simulink model "InversorTrifasico"  (R2022b)
settings: Solver=VariableStepAuto  StartTime=0.0  StopTime=3  MaxStep=0.00001  RelTol=1e-3
libraries: spsIGBTDiodeLib x6, spsVoltageMeasurementLib x3, spsSeriesRLCBranchLib x3, spsMeanLib x2, spsRMSLib x2, spsDCVoltageSourceLib x1, sps_lib x1
settings Model: Creator=mique  LastModifiedBy=ramuj

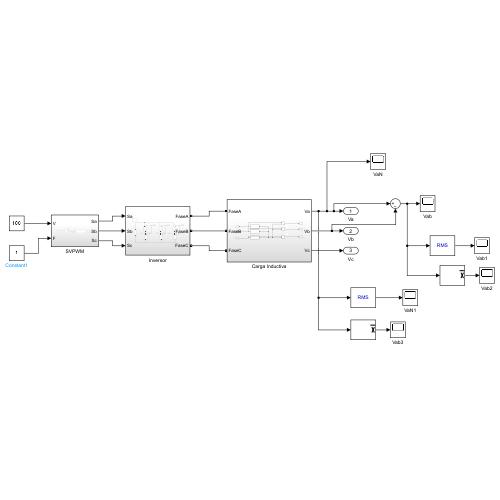
[thumbnail: Simulink's stored preview of the top-level diagram]
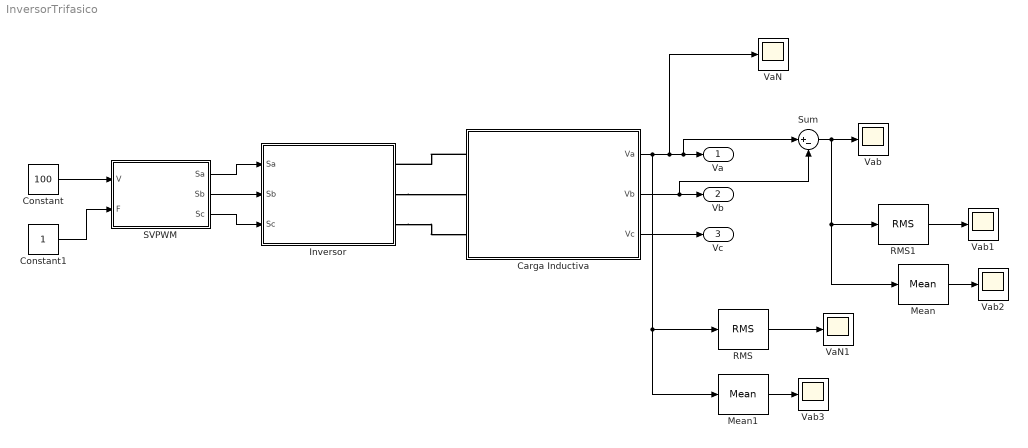
== system InversorTrifasico ==
  Carga Inductiva : Subsystem
  Constant : Constant  Value=100
  Constant1 : Constant
  Inversor : Subsystem
  Mean : spsMeanLib/Mean  Freq=60  Vinit=0  Ts=0
  Mean1 : spsMeanLib/Mean  Freq=60  Vinit=0  Ts=0
  RMS : spsRMSLib/RMS  TrueRMS=on  Freq=60  RMSInit=120  Ts=0
  RMS1 : spsRMSLib/RMS  TrueRMS=on  Freq=60  RMSInit=120  Ts=0
  SVPWM : Subsystem
  Sum : Sum  Inputs=|+-
  VaN : Scope
  VaN1 : Scope
  Vab{,1..3} (4 alike) : Scope
  Va : Outport
  Vb : Outport  Port=2
  Vc : Outport  Port=3
  wires:
  Carga Inductiva/2(Vb) -> Sum/2, Vb/1
  Carga Inductiva/3(Vc) -> Vc/1
  SVPWM/1(Sa) -> Inversor/1(Sa)
  SVPWM/2(Sb) -> Inversor/2(Sb)
  SVPWM/3(Sc) -> Inversor/3(Sc)
  Constant/1 -> SVPWM/1(V)
  Constant1/1 -> SVPWM/2(F)
  Sum/1 -> Mean/1, RMS1/1, Vab/1
  RMS/1 -> VaN1/1
  RMS1/1 -> Vab1/1
  Mean/1 -> Vab2/1
  Carga Inductiva/1(Va) -> Mean1/1, RMS/1, VaN/1, Sum/1, Va/1
  Mean1/1 -> Vab3/1
  connections:
  Carga Inductiva/LConn1 -- Inversor/RConn1
  Inversor/RConn2 -- Carga Inductiva/LConn2
  Inversor/RConn3 -- Carga Inductiva/LConn3

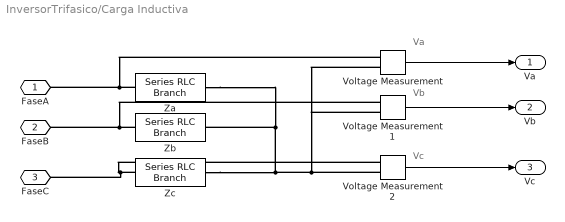
== system InversorTrifasico/Carga Inductiva ==
  note: Va
  note: Vb
  note: Vc
  Voltage Measurement : spsVoltageMeasurementLib/Voltage Measurement  PhasorSimulation=off  OutputType=Complex  PSBequivalent=0
  Voltage Measurement1 : spsVoltageMeasurementLib/Voltage Measurement  PhasorSimulation=off  OutputType=Complex  PSBequivalent=0
  Voltage Measurement2 : spsVoltageMeasurementLib/Voltage Measurement  PhasorSimulation=off  OutputType=Complex  PSBequivalent=0
  Za : spsSeriesRLCBranchLib/Series RLC Branch  LConnTagsString=__new0  RConnTagsString=__new0  BranchType=RL  Resistance=1e-3  Inductance=21e-3  SetiL0=off  InitialCurrent=0  Capacitance=1e-6  Setx0=off  InitialVoltage=0  Measurements=None
  Zb : spsSeriesRLCBranchLib/Series RLC Branch  LConnTagsString=__new0  RConnTagsString=__new0  BranchType=RL  Resistance=1e-3  Inductance=21e-3  SetiL0=off  InitialCurrent=0  Capacitance=1e-6  Setx0=off  InitialVoltage=0  Measurements=None
  Zc : spsSeriesRLCBranchLib/Series RLC Branch  LConnTagsString=__new0  RConnTagsString=__new0  BranchType=RL  Resistance=1e-3  Inductance=21e-3  SetiL0=off  InitialCurrent=0  Capacitance=1e-6  Setx0=off  InitialVoltage=0  Measurements=None
  FaseA : PMIOPort  Side=Left
  FaseB : PMIOPort  Port=2  Side=Left
  FaseC : PMIOPort  Port=3  Side=Left
  Va : Outport
  Vb : Outport  Port=2
  Vc : Outport  Port=3
  wires:
  Voltage Measurement/1 -> Va/1
  Voltage Measurement1/1 -> Vb/1
  Voltage Measurement2/1 -> Vc/1
  connections:
  Voltage Measurement1/LConn1 -- FaseB/RConn1 -- Zb/LConn1
  Voltage Measurement/LConn1 -- Za/LConn1 -- FaseA/RConn1
  Zc/RConn1 -- Voltage Measurement1/LConn2 -- Voltage Measurement/LConn2 -- Voltage Measurement2/LConn2 -- Za/RConn1 -- Zb/RConn1
  Voltage Measurement2/LConn1 -- Zc/LConn1 -- FaseC/RConn1

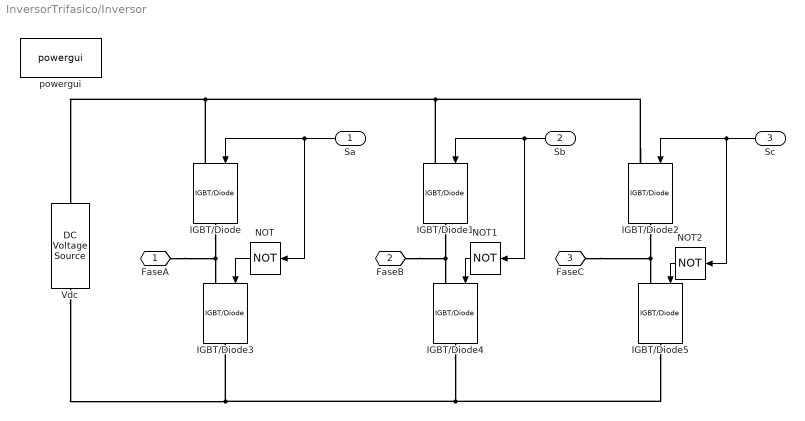
== system InversorTrifasico/Inversor ==
  Sa : Inport
  Sb : Inport  Port=2
  Sc : Inport  Port=3
  IGBT/Diode{,1..5} (6 alike) : spsIGBTDiodeLib/IGBT//Diode  Ron=1e-3  Rs=1e5  Cs=inf  Measurements=off
  NOT : Logic  Operator=NOT  IconShape=distinctive  AllPortsSameDT=off  OutDataTypeStr=boolean
  NOT1 : Logic  Operator=NOT  IconShape=distinctive  AllPortsSameDT=off  OutDataTypeStr=boolean
  NOT2 : Logic  Operator=NOT  IconShape=distinctive  AllPortsSameDT=off  OutDataTypeStr=boolean
  Vdc : spsDCVoltageSourceLib/DC Voltage Source  Amplitude=200  Measurements=None
  powergui : sps_lib/powergui  Priority=1  SimulationMode=Continuous  SampleTime=50e-6  frequency=60  Iterations=50  frequencyindice=0  Pbase=100e6  ErrMax=1e-4  UnitsV=kV  UnitsW=MW  buscounter=0  FunctionMessages=off  echomessages=off  EnableUseOfTLC=off  CurrentSourceSwitches=off  DisableSnubberDevices=off  DisableRonSwitches=off  DisableVfSwitches=off  DisplayEquations=off  AutomaticDiscreteSolvers=off  SolverType=Tustin/Backward Euler (TBE)  Interpol=off  ExternalGateDelay=off  methode=off  Ts=100  x0status=blocks  SPID=on  SwTol=0  HookPort=off  NonlinearTolerance=1e-4  nMaxIteration=100  ContinueOnMaxIteration=off  RestoreLinks=warning  ResistiveCurrentMeasurement=off  Frange=[0:2:500]  Ylog=off  Xlog=on  ShowGrid=off  save=off  variable=ZData  structure=0  ZoomFFT=off  StartTime=0.0  cycles=1  DisplayStyle=1  fundamental=60  FreqAxis=off  MaxFrequency=1000  frequencyindicesteady=1  RmsSteady=1  display=off
  FaseA : PMIOPort  Side=Right
  FaseB : PMIOPort  Port=2  Side=Right
  FaseC : PMIOPort  Port=3  Side=Right
  wires:
  Sa/1 -> IGBT/Diode/1, NOT/1
  NOT1/1 -> IGBT/Diode4/1
  Sb/1 -> IGBT/Diode1/1, NOT1/1
  NOT2/1 -> IGBT/Diode5/1
  Sc/1 -> IGBT/Diode2/1, NOT2/1
  NOT/1 -> IGBT/Diode3/1
  connections:
  Vdc/LConn1 -- IGBT/Diode3/RConn1 -- IGBT/Diode4/RConn1 -- IGBT/Diode5/RConn1
  IGBT/Diode2/RConn1 -- FaseC/RConn1 -- IGBT/Diode5/LConn1
  IGBT/Diode/LConn1 -- IGBT/Diode2/LConn1 -- IGBT/Diode1/LConn1 -- Vdc/RConn1
  IGBT/Diode/RConn1 -- FaseA/RConn1 -- IGBT/Diode3/LConn1
  IGBT/Diode1/RConn1 -- FaseB/RConn1 -- IGBT/Diode4/LConn1

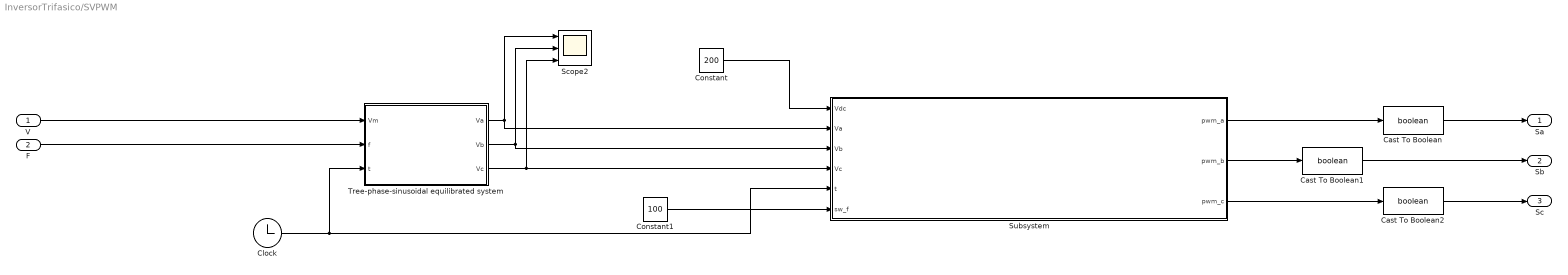
== system InversorTrifasico/SVPWM ==
  V : Inport
  F : Inport  Port=2
  Cast To Boolean : DataTypeConversion  OutDataTypeStr=boolean  SaturateOnIntegerOverflow=off  RndMeth=Floor
  Cast To Boolean1 : DataTypeConversion  OutDataTypeStr=boolean  SaturateOnIntegerOverflow=off  RndMeth=Floor
  Cast To Boolean2 : DataTypeConversion  OutDataTypeStr=boolean  SaturateOnIntegerOverflow=off  RndMeth=Floor
  Clock : Clock
  Constant : Constant  Value=200
  Constant1 : Constant  Value=100
  Scope2 : Scope  NumInputPorts=3
  Subsystem : Subsystem
  Tree-phase-sinusoidal equilibrated system : Subsystem
  Sa : Outport
  Sb : Outport  Port=2
  Sc : Outport  Port=3
  wires:
  Subsystem/1(pwm_a) -> Cast To Boolean/1
  Tree-phase-sinusoidal equilibrated system/3(Vc) -> Scope2/3, Subsystem/4(Vc)
  V/1 -> Tree-phase-sinusoidal equilibrated system/1(Vm)
  Subsystem/2(pwm_b) -> Cast To Boolean1/1
  F/1 -> Tree-phase-sinusoidal equilibrated system/2(f)
  Constant1/1 -> Subsystem/6(sw_f)
  Subsystem/3(pwm_c) -> Cast To Boolean2/1
  Clock/1 -> Tree-phase-sinusoidal equilibrated system/3(t), Subsystem/5(t)
  Tree-phase-sinusoidal equilibrated system/2(Vb) -> Scope2/2, Subsystem/3(Vb)
  Tree-phase-sinusoidal equilibrated system/1(Va) -> Scope2/1, Subsystem/2(Va)
  Cast To Boolean/1 -> Sa/1
  Cast To Boolean1/1 -> Sb/1
  Constant/1 -> Subsystem/1(Vdc)
  Cast To Boolean2/1 -> Sc/1

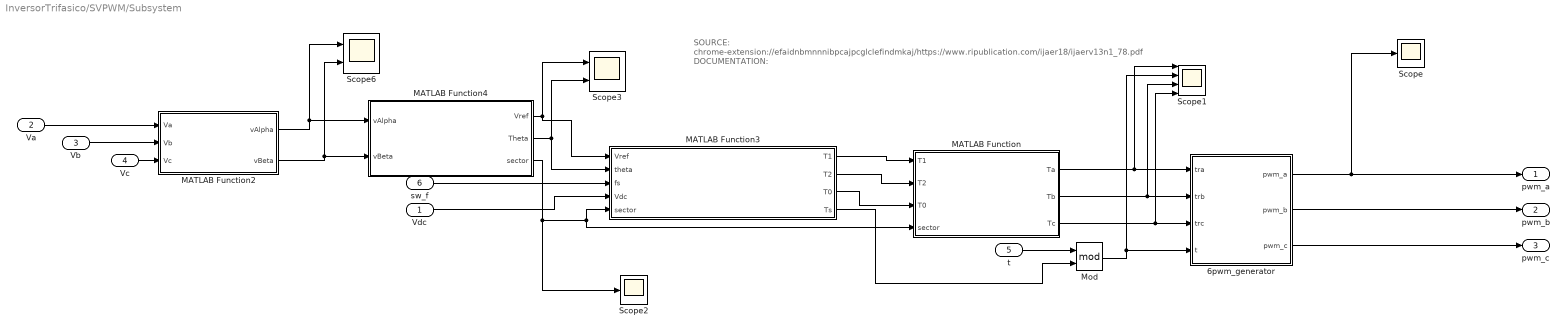
== system InversorTrifasico/SVPWM/Subsystem ==
  note: SOURCE:
      | chrome-extension://efaidnbmnnnibpcajpcglclefindmkaj/https://www.ripublication.com/ijaer18/ijaerv13n1_78.pdf
      | DOCUMENTATION:
  Vdc : Inport
  Va : Inport  Port=2
  Vb : Inport  Port=3
  Vc : Inport  Port=4
  t : Inport  Port=5
  sw_f : Inport  Port=6
  6pwm_generator : Subsystem
  MATLAB Function : MATLAB Function  TreatAsAtomicUnit=on
  MATLAB Function2 : MATLAB Function  TreatAsAtomicUnit=on
  MATLAB Function3 : MATLAB Function  TreatAsAtomicUnit=on
  MATLAB Function4 : MATLAB Function  TreatAsAtomicUnit=on
  Mod : Math  Operator=mod
  Scope : Scope
  Scope1 : Scope  NumInputPorts=4
  Scope2 : Scope
  Scope3 : Scope  NumInputPorts=2
  Scope6 : Scope  NumInputPorts=2
  pwm_a : Outport
  pwm_b : Outport  Port=2
  pwm_c : Outport  Port=3
  wires:
  MATLAB Function4/3(sector) -> Scope2/1, MATLAB Function/4(sector), MATLAB Function3/5(sector)
  MATLAB Function3/1(T1) -> MATLAB Function/1(T1)
  MATLAB Function2/2(vBeta) -> Scope6/2, MATLAB Function4/2(vBeta)
  MATLAB Function4/2(Theta) -> MATLAB Function3/2(theta), Scope3/2
  MATLAB Function4/1(Vref) -> MATLAB Function3/1(Vref), Scope3/1
  MATLAB Function3/3(T0) -> MATLAB Function/3(T0)
  MATLAB Function3/2(T2) -> MATLAB Function/2(T2)
  Vdc/1 -> MATLAB Function3/4(Vdc)
  MATLAB Function2/1(vAlpha) -> MATLAB Function4/1(vAlpha), Scope6/1
  MATLAB Function/2(Tb) -> Scope1/3, 6pwm_generator/2(trb)
  6pwm_generator/3(pwm_c) -> pwm_c/1
  MATLAB Function/1(Ta) -> Scope1/1, 6pwm_generator/1(tra)
  sw_f/1 -> MATLAB Function3/3(fs)
  MATLAB Function/3(Tc) -> Scope1/4, 6pwm_generator/3(trc)
  Vb/1 -> MATLAB Function2/2(Vb)
  Va/1 -> MATLAB Function2/1(Va)
  Vc/1 -> MATLAB Function2/3(Vc)
  6pwm_generator/1(pwm_a) -> Scope/1, pwm_a/1
  6pwm_generator/2(pwm_b) -> pwm_b/1
  t/1 -> Mod/1
  Mod/1 -> Scope1/2, 6pwm_generator/4(t)
  MATLAB Function3/4(Ts) -> Mod/2

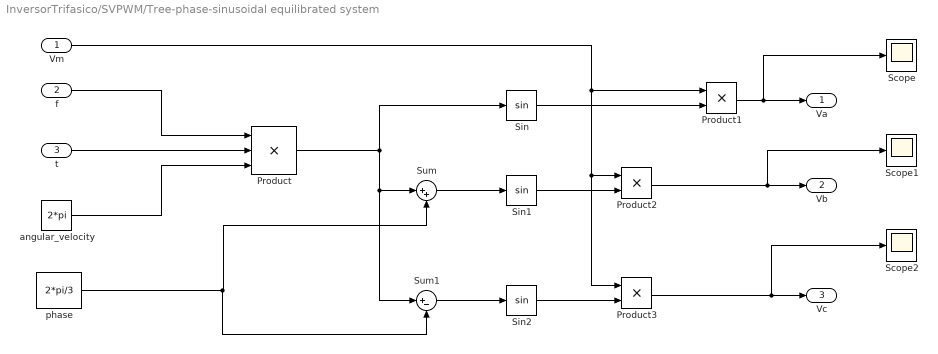
== system InversorTrifasico/SVPWM/Tree-phase-sinusoidal equilibrated system ==
  Vm : Inport
  f : Inport  Port=2
  t : Inport  Port=3
  Product : Product  Inputs=3
  Product1 : Product
  Product2 : Product
  Product3 : Product
  Scope : Scope
  Scope1 : Scope
  Scope2 : Scope
  Sin : Trigonometry
  Sin1 : Trigonometry
  Sin2 : Trigonometry
  Sum : Sum  Inputs=|++
  Sum1 : Sum  Inputs=|+-
  angular_velocity : Constant  Value=2*pi
  phase : Constant  Value=2*pi/3
  Va : Outport
  Vb : Outport  Port=2
  Vc : Outport  Port=3
  wires:
  f/1 -> Product/1
  t/1 -> Product/2
  angular_velocity/1 -> Product/3
  Product/1 -> Sin/1, Sum/1, Sum1/1
  Vm/1 -> Product3/1, Product2/1, Product1/1
  Sin/1 -> Product1/2
  Product1/1 -> Scope/1, Va/1
  phase/1 -> Sum1/2, Sum/2
  Sum/1 -> Sin1/1
  Sin1/1 -> Product2/2
  Product2/1 -> Scope1/1, Vb/1
  Sum1/1 -> Sin2/1
  Sin2/1 -> Product3/2
  Product3/1 -> Scope2/1, Vc/1

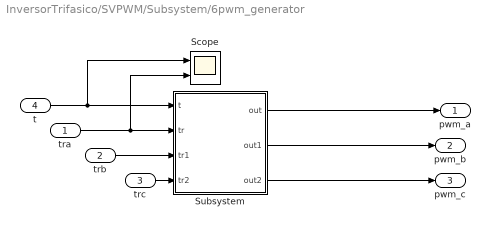
== system InversorTrifasico/SVPWM/Subsystem/6pwm_generator ==
  tra : Inport
  trb : Inport  Port=2
  trc : Inport  Port=3
  t : Inport  Port=4
  Scope : Scope  NumInputPorts=2
  Subsystem : Subsystem
  pwm_a : Outport
  pwm_b : Outport  Port=2
  pwm_c : Outport  Port=3
  wires:
  Subsystem/2(out1) -> pwm_b/1
  Subsystem/3(out2) -> pwm_c/1
  Subsystem/1(out) -> pwm_a/1
  tra/1 -> Scope/2, Subsystem/2(tr)
  trc/1 -> Subsystem/4(tr2)
  trb/1 -> Subsystem/3(tr1)
  t/1 -> Scope/1, Subsystem/1(t)

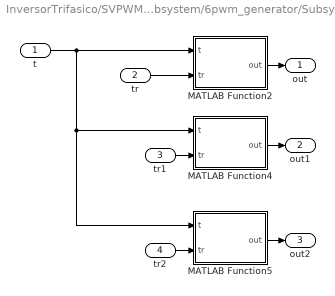
== system InversorTrifasico/SVPWM/Subsystem/6pwm_generator/Subsystem ==
  t : Inport
  tr : Inport  Port=2
  tr1 : Inport  Port=3
  tr2 : Inport  Port=4
  MATLAB Function2 : MATLAB Function  TreatAsAtomicUnit=on
  MATLAB Function4 : MATLAB Function  TreatAsAtomicUnit=on
  MATLAB Function5 : MATLAB Function  TreatAsAtomicUnit=on
  out : Outport
  out1 : Outport  Port=2
  out2 : Outport  Port=3
  wires:
  MATLAB Function4/1(out) -> out1/1
  tr2/1 -> MATLAB Function5/2(tr)
  tr1/1 -> MATLAB Function4/2(tr)
  tr/1 -> MATLAB Function2/2(tr)
  MATLAB Function2/1(out) -> out/1
  t/1 -> MATLAB Function5/1(t), MATLAB Function4/1(t), MATLAB Function2/1(t)
  MATLAB Function5/1(out) -> out2/1

== matlab function InversorTrifasico/SVPWM/Subsystem/MATLAB Function ==
  data: T1 input; T2 input; T0 input; Ta output; sector input; Tb output; Tc output
function [Ta, Tb, Tc] = switches(T1, T2, T0, sector)
switch sector
    case 1
        Ta = T1 + T2 + T0/2;
        Tb = T2 + T0/2;
        Tc = T0/2;
    case 2
        Ta = T1 + T0/2;
        Tb = T1 + T2 + T0/2;
        Tc = T0/2;
    case 3
        Ta = T0/2;
        Tb = T1 + T2 + T0/2;
        Tc = T2 + T0/2;
    case 4
        Ta = T0/2;
        Tb = T1 + T0/2;
        Tc = T1 + T2 + T0/2;
    case 5
        Ta = T2 + T0/2;
        Tb = T0/2;
        Tc = T1 + T2 + T0/2;
    case 6
        Ta = T1 + T2 + T0/2;
        Tb = T0/2;
        Tc = T1 + T0/2;
    otherwise
        Ta = 0;
        Tb = 0;
        Tc = 0;
end

== matlab function InversorTrifasico/SVPWM/Subsystem/MATLAB Function3 ==
  data: Vref input; T1 output; theta input; T2 output; T0 output; fs input; Vdc input; sector input; Ts output
function [T1, T2, T0,Ts] = times(Vref, theta, fs, Vdc, sector)

Ts = 1/fs;

T1 = (sqrt(3)*Ts*abs(Vref))/Vdc * sin((sector/3)*pi-theta);
T2 = (sqrt(3)*Ts*abs(Vref))/Vdc * sin(theta - ((sector-1)/3)*pi);


T0 = Ts - (T1 + T2);

== matlab function InversorTrifasico/SVPWM/Subsystem/6pwm_generator/Subsystem/MATLAB Function2 ==
  data: t input; out output; tr input
function out = pwm(t,tr)
if t>=tr
    out = 0;
else 
    out = 1;
end

== matlab function InversorTrifasico/SVPWM/Subsystem/6pwm_generator/Subsystem/MATLAB Function4 ==
  data: t input; out output; tr input
function out = pwm(t,tr)
if t>=tr
    out = 0;
else 
    out = 1;
end

== matlab function InversorTrifasico/SVPWM/Subsystem/6pwm_generator/Subsystem/MATLAB Function5 ==
  data: t input; out output; tr input
function out = pwm(t,tr)
if t>=tr
    out = 0;
else 
    out = 1;
end

== matlab function InversorTrifasico/SVPWM/Subsystem/MATLAB Function2 ==
  data: Va input; vAlpha output; Vb input; vBeta output; Vc input
function [vAlpha,vBeta] = alpha_beta(Va, Vb, Vc)
vAlpha = (2/3)*Va - (1/3)*Vb - (1/3)*Vc;
vBeta = (sqrt(3)/3)*Vb - (sqrt(3)/3)*Vc;

end

== matlab function InversorTrifasico/SVPWM/Subsystem/MATLAB Function4 ==
  data: vAlpha input; Vref output; vBeta input; Theta output; sector output
function [Vref,Theta, sector] = generate_vref_theta(vAlpha, vBeta)
  Vref = sqrt((vAlpha^2) + (vBeta^2));
  Theta = atan2(vBeta, vAlpha);

if(Theta>0 && Theta<60/180*pi)
    sector=1;
elseif(Theta>60/180*pi && Theta<120/180*pi)
    sector=2;
elseif(Theta>120/180*pi && Theta<180/180*pi)
    sector=3;
elseif(Theta>-180/180*pi && Theta<-120/180*pi)
    sector=4;
elseif(Theta>-120/180*pi && Theta<-60/180*pi)
    sector=5;
elseif(Theta>-60/180*pi && Theta<0/180*pi)
    sector=6;    
else
    sector=0;
end
